simulink model "InvertedPendulumRobot_MPC_Controller"  (R2024b)
settings: configuration reference "controller_config" (kept outside this file)
values from neighbouring files (symbols this model uses):
  TimeStep = 0.01    [InvertedPendulumRobot_data.sldd]
undefined symbols (not defined in the file or in its folder): param, u0
libraries: mpclib x1
settings Model: DataDictionary=InvertedPendulumRobot_data.sldd  Creator=tshintai  LastModifiedBy=tshintai
settings ConfigSetRef: SourceName=controller_config

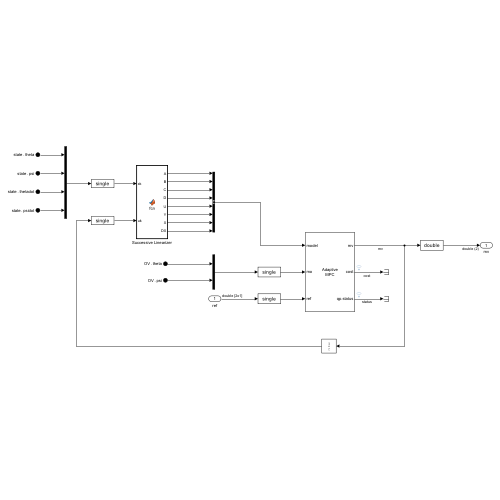
[thumbnail: Simulink's stored preview of the top-level diagram]
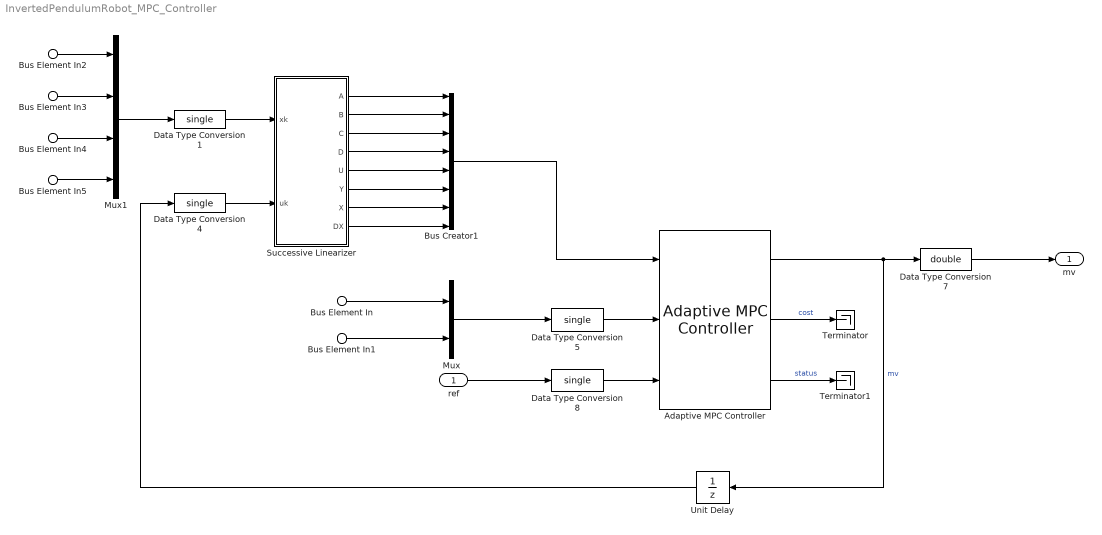
== system InvertedPendulumRobot_MPC_Controller ==
  ref : Inport  OutDataTypeStr=double  PortDimensions=[2 1]
  Bus Element In : Inport  Port=2  PortName=OV  Element=theta
  Bus Element In1 : Inport  Port=2  PortName=OV  Element=psi
  Bus Element In2 : Inport  Port=3  PortName=state  Element=theta
  Bus Element In3 : Inport  Port=3  PortName=state  Element=psi
  Bus Element In4 : Inport  Port=3  PortName=state  Element=thetadot
  Bus Element In5 : Inport  Port=3  PortName=state  Element=psidot
  Adaptive MPC Controller : mpclib/Adaptive MPC Controller  SCDEnableBlockLinearizationSpecification=on  mpcobj=mpcobj  x0=stateobj  enable_value=0  updateMPCinCallerWorkspace=on  md_inport=off  mv_inport=off  uref_inport=off  return_cost=on  return_mvseq=off  return_qpstatus=on  return_xseq=off  return_state=off  return_ovseq=off  state_inport=off  isltv_plant=off  umin_inport=off  umax_inport=off  ymin_inport=off  ymax_inport=off  cc_inport=off  ywt_inport=off  uwt_inport=off  duwt_inport=off  rhoeps_inport=off  pm_inport=off  MaximumP=10  HorizonChoice=FixedHorizon  BlockDataType=single  SampleTimeInherited=off  switch_inport=off
  Bus Creator1 : BusCreator  Inputs=8
  Data Type Conversion{1,4..5,8} (4 alike) : DataTypeConversion  OutDataTypeStr=single  SaturateOnIntegerOverflow=off  RndMeth=Floor
  Data Type Conversion7 : DataTypeConversion  OutDataTypeStr=double  SaturateOnIntegerOverflow=off  RndMeth=Floor
  Mux : Mux  Inputs=2
  Mux1 : Mux
  Successive Linearizer : MATLAB Function  TreatAsAtomicUnit=on
  Terminator : Terminator
  Terminator1 : Terminator
  Unit Delay : UnitDelay  InitialCondition=u0  SampleTime=-1  HasFrameUpgradeWarning=on
  mv : Outport  OutDataTypeStr=double  PortDimensions=2
  wires:
  Bus Element In3/1 -> Mux1/2
  Successive Linearizer/6(Y) -> Bus Creator1/6
  Bus Element In1/1 -> Mux/2
  Bus Element In2/1 -> Mux1/1
  Mux1/1 -> Data Type Conversion1/1
  Data Type Conversion1/1 -> Successive Linearizer/1(xk)
  Bus Creator1/1 -> Adaptive MPC Controller/1
  Successive Linearizer/8(DX) -> Bus Creator1/8
  ref/1 -> Data Type Conversion8/1
  Successive Linearizer/2(B) -> Bus Creator1/2
  Data Type Conversion4/1 -> Successive Linearizer/2(uk)
  Successive Linearizer/4(D) -> Bus Creator1/4
  Successive Linearizer/1(A) -> Bus Creator1/1
  Data Type Conversion8/1 -> Adaptive MPC Controller/3
  Successive Linearizer/5(U) -> Bus Creator1/5
  Adaptive MPC Controller/2 -> Terminator/1  "cost"
  Mux/1 -> Data Type Conversion5/1
  Bus Element In/1 -> Mux/1
  Data Type Conversion7/1 -> mv/1
  Successive Linearizer/3(C) -> Bus Creator1/3
  Data Type Conversion5/1 -> Adaptive MPC Controller/2
  Unit Delay/1 -> Data Type Conversion4/1
  Adaptive MPC Controller/3 -> Terminator1/1  "status"
  Adaptive MPC Controller/1 -> Unit Delay/1, Data Type Conversion7/1  "mv"
  Bus Element In4/1 -> Mux1/3
  Successive Linearizer/7(X) -> Bus Creator1/7
  Bus Element In5/1 -> Mux1/4

== matlab function InvertedPendulumRobot_MPC_Controller/Successive Linearizer ==
  settings: sampleTime=Ts
  data: xk input; uk input; A output; B output; C output; D output; U output size=[2,1]; Y output size=[2,1]; X output size=[4,1]; DX output size=[4,1]; TimeStep parameter; param parameter
function [A,B,C,D,U,Y,X,DX] = fcn(xk,uk,TimeStep,param)
% Order of state, input and output
nx = cast(4, 'like', xk);
nu = cast(2, 'like', xk);
ny = cast(2, 'like', xk);
% Initialize outputs
A = zeros(nx,nx, 'like', xk);
B = zeros(nx,nu, 'like', xk);
C = zeros(ny,nx, 'like', xk);
D = zeros(ny,nu, 'like', xk);
U = zeros(nu,1, 'like', xk);
Y = zeros(ny,1, 'like', xk);
X = zeros(nx,1, 'like', xk);
DX = zeros(nx,1, 'like', xk);
% Obtain time invarying linear models via successive linearization
% analytical linearization (continuous time)
[DXk, yk, Ak, Bk0, Ck, Dk] = InvertedPendulumRobot_CT(xk, uk, param);
% append dx offset 
Bk = [Bk0 DXk];
% convert A and B matrices from continuous time to discrete time
[Ak, Bk] = getDiscrete(Ak, Bk, cast(TimeStep, 'like', xk));
% obtain matrices
A = Ak;
B = Bk(:,1:nu);
C = Ck;
D = Dk;
U = uk;
Y = yk;
X = xk;
DX = Bk(:,nu+1);

end

function [A, B] = getDiscrete(a, b, Ts)
% Convert A, B to discrete time
A = expm(a*Ts);
nx = size(b,1);
n = 4;  % Number of points for Simpson's Rule, an even integer >= 2.
% Use Simpson's rule to compute integral(0,Ts){expm(a*s)*ds*b}
h = Ts/n;
Ai = eye(nx, 'like', b) + A;        % First and last terms;
Coef = 2;
for i = 1:n-1
    if Coef == 2
        Coef = 4;
    else
        Coef = 2;
    end
    Ai = Ai + Coef*expm(a*i*h);     % Intermediate terms
end
B = cast(h/3, 'like', b)*Ai*b;
end
